simulink model "Feedforward"  (R2025b)
settings: Solver=VariableStepAuto  StartTime=0.0  StopTime=500  RelTol=1e-3
settings Model: Creator=denni  LastModifiedBy=hakee
settings RTWCC: GPUComputeCapability=3.5

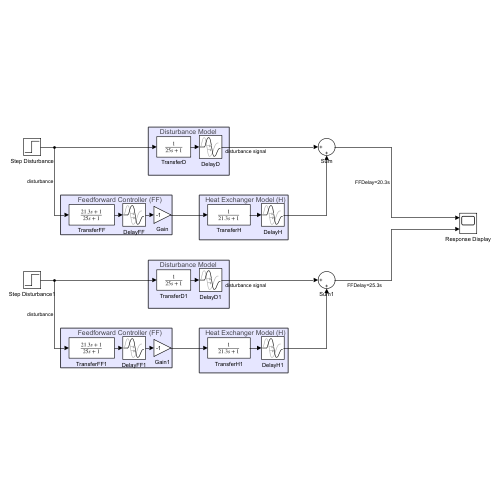
[thumbnail: Simulink's stored preview of the top-level diagram]
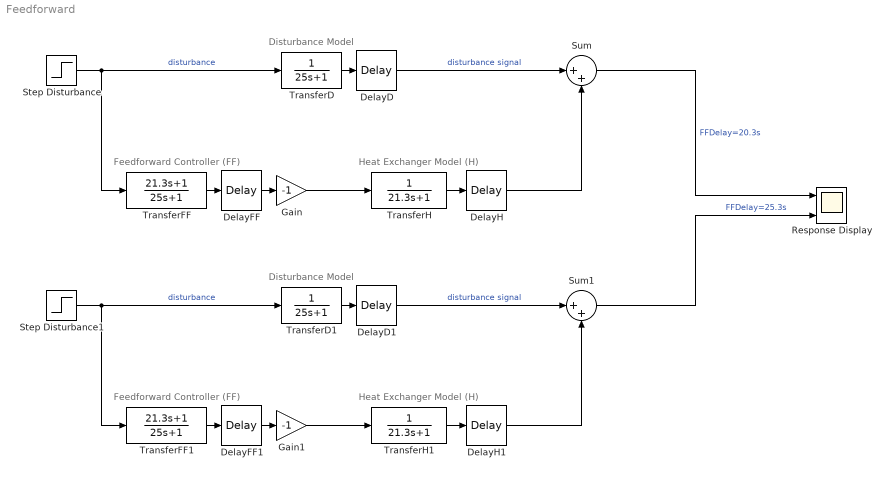
== system Feedforward ==
  note: Feedforward Controller (FF)
  note: Heat Exchanger Model (H)
  note: Disturbance Model
  note: Feedforward Controller (FF)
  note: Heat Exchanger Model (H)
  note: Disturbance Model
  DelayD : TransportDelay  DelayTime=35
  DelayD1 : TransportDelay  DelayTime=35
  DelayFF : TransportDelay  DelayTime=20.3
  DelayFF1 : TransportDelay  DelayTime=25.3
  DelayH : TransportDelay  DelayTime=14.7
  DelayH1 : TransportDelay  DelayTime=14.7
  Gain : Gain  Gain=-1
  Gain1 : Gain  Gain=-1
  Response Display : Scope  NumInputPorts=2
      settings: ActiveDisplayYMinimum=-0.51850689271566752  ActiveDisplayYMaximum=2.1751996684004959
  Step Disturbance : Step  Time=0  SampleTime=0
  Step Disturbance1 : Step  Time=0  SampleTime=0
  Sum : Sum  Inputs=|++
  Sum1 : Sum  Inputs=|++
  TransferD : TransferFcn  Denominator=[25 1]  ContinuousStateAttributes='heat'
  TransferD1 : TransferFcn  Denominator=[25 1]  ContinuousStateAttributes='heat'
  TransferFF : TransferFcn  Numerator=[21.3 1]  Denominator=[25 1]  ContinuousStateAttributes='heat'
  TransferFF1 : TransferFcn  Numerator=[21.3 1]  Denominator=[25 1]  ContinuousStateAttributes='heat'
  TransferH : TransferFcn  Denominator=[21.3 1]  ContinuousStateAttributes='heat'
  TransferH1 : TransferFcn  Denominator=[21.3 1]  ContinuousStateAttributes='heat'
  wires:
  TransferD/1 -> DelayD/1
  Sum/1 -> Response Display/1  "FFDelay=20.3s"
  DelayFF/1 -> Gain/1
  TransferFF/1 -> DelayFF/1
  DelayD/1 -> Sum/1  "disturbance signal"
  Step Disturbance/1 -> TransferD/1, TransferFF/1  "disturbance"
  TransferH/1 -> DelayH/1
  DelayH/1 -> Sum/2
  Gain/1 -> TransferH/1
  DelayD1/1 -> Sum1/1  "disturbance signal"
  Step Disturbance1/1 -> TransferD1/1, TransferFF1/1  "disturbance"
  DelayH1/1 -> Sum1/2
  Gain1/1 -> TransferH1/1
  Sum1/1 -> Response Display/2  "FFDelay=25.3s"
  TransferD1/1 -> DelayD1/1
  TransferH1/1 -> DelayH1/1
  TransferFF1/1 -> DelayFF1/1
  DelayFF1/1 -> Gain1/1
